simulink model "PhyMtrCtrl"  (R2023b)
settings: Solver=VariableStepAuto  StartTime=0.0  StopTime=10.0  RelTol=1e-3
values from neighbouring files (symbols this model uses):
  B = 0.001889    [MtrCtrl_v01.sldd]    (also in PICal.m; PMSM.m = Simulink.Parameter)
  C_LUT_AngleTable_sng_Null = saveVarsMat.C_LUT_AngleTable_sng_Null    [AngleTable.m]    (also in PMSM.m)
  C_LUT_SinTable_sng_Null = saveVarsMat.C_LUT_SinTable_sng_Null    [AngleTable.m]    (also in PMSM.m)
  C_MATH_OneOverSqrtThree_s32n31_Null = Simulink.Parameter    [PMSM.m]
  C_MATH_Pi_u32n30_Null = Simulink.Parameter    [PMSM.m]
  C_MATH_SqrtThreeOverThree_s32n31_Null = Simulink.Parameter    [PMSM.m]
  C_PMSM_CurQKi_u32n31_null = Simulink.Parameter    [PMSM.m]
  C_PMSM_CurQKp_u32n31_null = Simulink.Parameter    [PMSM.m]
  C_PMSM_Flux_u32n32_Vs = Simulink.Parameter    [PMSM.m]
  Flux = 0.192    [MtrCtrl_v01.sldd]    (also in PICal.m; PMSM.m)
  IBase_A = 2000.0    [MtrCtrl_v01.sldd]    (also in PICal.m = 300; PMSM.m = Simulink.Parameter)
  J = 0.011    [MtrCtrl_v01.sldd]    (also in PICal.m; PMSM.m)
  K_SVM_DefultDuty_s32n31_Null = Simulink.Parameter    [PMSM.m]
  KCCM_VirPosn_flg = 0.0    [MtrCtrl_v01.sldd]    (also in PMSM.m = Simulink.Parameter)
  KCCM_VoltModeEna_Flg = 0.0    [MtrCtrl_v01.sldd]    (also in PMSM.m = Simulink.Parameter)
  Kis = 114583.3333333333    [MtrCtrl_v01.sldd]    (also in PICal.m = 114583.333333; PMSM.m = 114583.333333)
  Kt = 1.1520000000000001    [MtrCtrl_v01.sldd]    (also in PICal.m = 1.152; PMSM.m = 1.152)
  Ld = 80e-6    (= 8e-05)    [FluxweakingGen.m]    (also in IEHB_MAPGenerationtest.m = 6.8e-05; MtrCtrl_v01.sldd = 0.000635; PICal.m = 0.000635; PMSM.m = Simulink.Parameter)
  LPF_coefg = 0.01    [MtrCtrl_v01.sldd]    (also in PMSM.m = Simulink.Parameter)
  Lq = 80e-6    (= 8e-05)    [FluxweakingGen.m]    (also in IEHB_MAPGenerationtest.m = 6e-05; MtrCtrl_v01.sldd = 0.000685; PICal.m = 0.000635; PMSM.m = Simulink.Parameter)
  Ls = 0.000635    [MtrCtrl_v01.sldd]    (also in PICal.m; PMSM.m)
  OneOverUBase_V = Simulink.Parameter    [PMSM.m]
  Pp = 4.0    [MtrCtrl_v01.sldd]    (also in PICal.m = 4; PMSM.m = Simulink.Parameter)
  Rs = 0.03    [FluxweakingGen.m]    (also in MtrCtrl_v01.sldd = 0.05; PICal.m = 0.05; PMSM.m = Simulink.Parameter)
  SecPerRnd = 0.6    [MtrCtrl_v01.sldd]    (also in PMSM.m = Simulink.Parameter)
  sinTable = 0.0015339801862847655 0.0015339807878856412 0.0030679567629659761 0.0030679615757712823 0.0046019261204485705 0.0046019423636569235 0.0061358846491544753 0.0061359231515425647 0.007669828739531097 0.0076699039394282058 0.00920375478205982 0.009203884727313847 0.010737659167264491 0.010737865515199488 0.012271538285719925 0.012271846303085129 0.013805388528060391 0.013805827090970771 0.015339206284    [MtrCtrl_v01.sldd]    (also in SinLut.m = zeros(2,TableSize))
  SMOGain_V = 323.31615074619043    [MtrCtrl_v01.sldd]    (also in PMSM.m = Simulink.Parameter)
  Ts = 0.0001    [MtrCtrl_v01.sldd]    (also in PICal.m; PMSM.m = Simulink.Parameter)
  UBase_V = 600.0    [MtrCtrl_v01.sldd]    (also in PICal.m = 600; PMSM.m = Simulink.Parameter)
  wmBase_rps = 314.15926535897933    [MtrCtrl_v01.sldd]    (also in PICal.m = 314.159265359; PMSM.m = Simulink.Parameter)
undefined symbols (not defined in the file or in its folder): C_PMSM_Ls_pu, C_PMSM_PolePairs_u8_Null, DiscIntNeverNeededParam
libraries: ee_lib x16, simulink x10, nesl_utility x6, spsVoltageMeasurementLib x6, spsCurrentMeasurementLib x3, spsSeriesRLCBranchLib x3, simulink_extras x2, fl_lib x2, sdl_lib x1, eePmsmFwController x1, slpidlib x1, spspowerguiLib x1
(part 1 of 3)
settings Model: Creator=z1486  LastModifiedBy=z1486

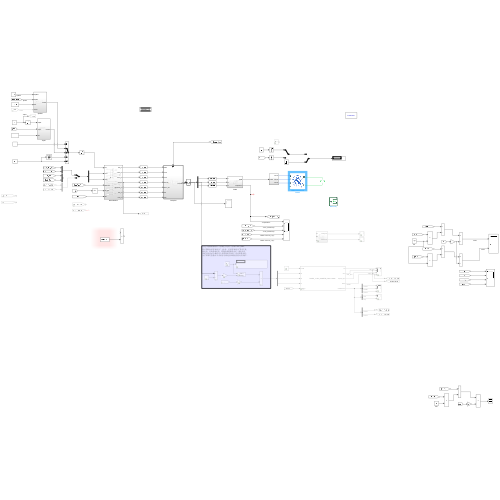
[thumbnail: Simulink's stored preview of the top-level diagram]
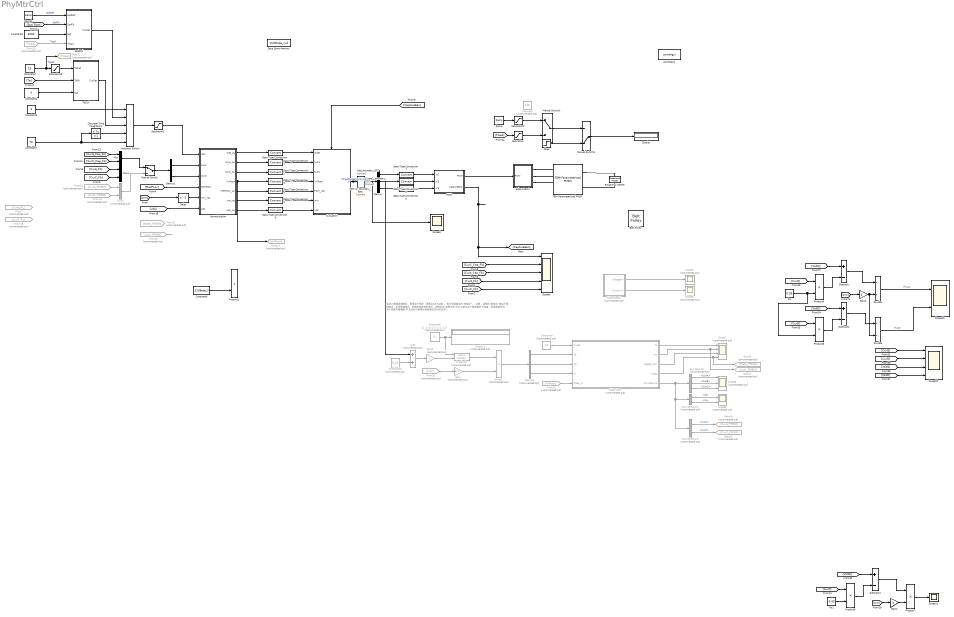
== system PhyMtrCtrl ==
  note: 经过三角载波调制后，再乘这个矩阵，再乘以1/3与Udc，
      | 即可得到真实的“相电压”。(注意，这里的“相电压”其实不是
      | 相电压，应该是端电压，即电机端到地的电压，相电压应
      | 该是正弦)为什么乘以这个矩阵暂时不知道，但结果是对的。
      | 关于结果可查看表“开关状态与相电压和线电压的对应关系”。
  Add : Sum  Commented=on
  Add_boundary_DTC : DataTypeConversion
  Belt Pulley : sdl_lib/Couplings & Drives/Belt Pulley  belt_type=sdl.enum.belt_type.ideal  sheave_ang=30 deg  num_belts=1  model_f_c=sdl.enum.model_centrifugal.off  linear_density=0.6 kg/m  belt_direction=sdl.enum.belt_direction.opposite  breakable=sdl.enum.max_tension.off  F_max=1e5 N  check_tension=sdl.enum.tension_check.off  pulley_moveable=simscape.enum.onoff.off  r_pulley=.15 m  b_pulley=0.001 N*m*s/rad  model_inertia=sdl.enum.model_inertia.off  pulley_mass=0.01 kg  initial_vel=0 m/s  pulley_inertia=0.01 kg*m^2  initial_velocity=0 rad/s  friction_model=sdl.enum.PulleyModel.Modal  initial_state_locked=sdl.enum.initial_lock.unlocked  mu=0.5  mu_static=0.5  mu_kinetic=0.42  phi_wrap=180 deg  v_thr=0.001 m/s  f_thr=0.01 N
      settings: InternalSimscapePortConfiguration="{\"Bottom\":[],\"Left\":[{\"id\":\"S\",\"label\":\"S\",\"type\":\"foundation.mechanical.rotational.rotational\"}],\"Right\":[{\"id\":\"A\",\"label\":\"A\",\"type\":\"foundation.mechanical.translational.translational\"},{\"id\":\"B\",\"label\":\"B\",\"type\":\"foundation.mechanical.translational.translational\"}],\"Top\":[]}"
  Bus Selector : BusSelector  Commented=on  OutputSignals=CurA,CurB,CurC
  Bus Selector2 : BusSelector  Commented=on  OutputSignals=Id,Iq
  Bus Selector3 : BusSelector  Commented=on  OutputSignals=CurA,CurC
  Constant : Constant  Commented=on  Value=100
  Constant10 : Constant  Commented=on  Value=0.25
  Constant2 : Constant  Value=15
  Constant3 : Constant  Value=3
  Constant4 : Constant  Value=5
  Constant5 : Constant  Value=3000
  Constant6 : Constant  Value=1/UBase_V
  Constant7 : Constant  Value=70
  Constant8 : Constant  Commented=on  Value=[2 -1 -1;-1 2 -1;-1 -1 2]
  Constant9 : Constant  Commented=on  Value=10
  CurLpCtrl : Subsystem
      settings: RTWSystemCode=Nonreusable function  RTWFcnNameOpts=Use subsystem name
  Data Store Memory : DataStoreMemory  DataStoreName=VoltMode_null  WriteAfterWriteMsg=warning  ShowAdditionalParam=off
  Data Type Conversion{,1..9} (10 alike) : DataTypeConversion  SaturateOnIntegerOverflow=off  RndMeth=Floor
  Delay : Delay  DelayLength=1
  Demux : Demux  Outputs=3
  Demux1 : Demux  Outputs=2
  Demux2 : Demux  Commented=on  Outputs=3
  Demux_boundary_DTC : DataTypeConversion
  Discrete-Time Integrator2 : DiscreteIntegrator  SampleTime=-1  ICPrevOutput=DiscIntNeverNeededParam  ICPrevScaledInput=DiscIntNeverNeededParam
  Display : Display
  Display1 : Display  Commented=on
  Divide1 : Product  Commented=on  Inputs=**
  Divide2 : Product  Inputs=*/
  Divide3 : Product  Inputs=*/
  FEM-Parameterized PMSM : ee_lib/Electromechanical/Permanent Magnet/FEM-Parameterized PMSM  parameterization=1  winding_type=ee.enum.statorconnection.wye  iVec=[-300, 0, 300] A  xVec=[0, 20, 40, 60] deg  dfluxdiMatrix=0.0002 * ones(3, 4) Wb/A  dfluxdxMatrix=[0, -.16, .16, 0; 0, -.16, .16, 0; 0, -.16, .16, 0] Wb/rad  calculate_torque_matrix=1  TorqueMatrix=zeros(3, 3, 3, 4) N*m  idVec1=[-200, 0, 200] A  iqVec1=[-200, 0, 200] A  LdMatrix=0.0002 * ones(3, 3) H  LqMatrix=0.0002 * ones(3, 3) H  PmMatrix=0.1 * ones(3, 3) Wb  N=4  interp_method=simscape.enum.interpolation.linear  Rs=0.05 Ohm  Ms=0.00002 H  L0=0.00016 H  loss_param=ee.enum.fem_motor.ironLosses.empirical  losses_oc=[0, 0, 0] W  losses_sc=[0, 0, 0] W  f_losses=60 Hz  Isc_losses=95 A  Inertia=0.01 kg*m^2  lam=0 N*m*s/rad  i_d_specify=off  i_d_priority=None  i_d=0 A  i_d_nominal_specify=off  i_d_nominal_unit=A  i_d_nominal_value=1  i_q_specify=off  i_q_priority=None  i_q=0 A  i_q_nominal_specify=off  i_q_nominal_unit=A  i_q_nominal_value=1  torque_specify=off  torque_priority=None  torque=0 N*m  torque_nominal_specify=off  torque_nominal_unit=N*m  torque_nominal_value=1  angular_velocity_specify=off  angular_velocity_priority=High  angular_velocity=0 rpm  angular_velocity_nominal_specify=off  angular_velocity_nominal_unit=rpm  angular_velocity_nominal_value=1  angular_position_specify=off  angular_position_priority=High  angular_position=0 deg  angular_position_nominal_specify=off  angular_position_nominal_unit=deg  angular_position_nominal_value=1  Tmeas=298.15 K  alpha=3.93e-3 1/K  alpha_flux=-0.001 1/K  stator_thermal_mass=100 J/K  stator_initial_temperatures=[298.15, 298.15, 298.15] K  rotor_thermal_mass=200 J/K  rotor_initial_temperature=298.15 K  Rm_percent_rotor=90  Rd_percent_rotor=30  idVec=[-200, 0, 200] A  iqVec=[-200, 0, 200] A  dfluxAdiaMatrix3D=zeros(3, 3, 4) Wb/A  dfluxAdibMatrix3D=zeros(3, 3, 4) Wb/A  dfluxAdicMatrix3D=zeros(3, 3, 4) Wb/A  dfluxAdxMatrix3D=zeros(3, 3, 4) Wb/rad  TorqueMatrix3D=zeros(3, 3, 4) N*m  iaVec=[-200, 0, 200] A  ibVec=[-200, 0, 200] A  icVec=[-200, 0, 200] A  dfluxAdiaMatrix=zeros(3, 3, 3, 4) Wb/A  dfluxAdibMatrix=zeros(3, 3, 3, 4) Wb/A  dfluxAdicMatrix=zeros(3, 3, 3, 4) Wb/A  dfluxAdxMatrix=zeros(3, 3, 3, 4) Wb/rad  param_dq0=ee.enum.fem_motor.fluxTabulationOption.DQcartesian  winding_type_dq0=ee.enum.statorconnection.wye  expose_neutral_port=ee.enum.fem_motor.exposeNeutralPort.no  nPolePairs=4  parks_type=ee.enum.fem_motor.parksType.QleadsD_AphaseToDaxis  idVec2=[-200, 0, 200] A  iqVec2=[-200, 0, 200] A  magVec2=[0, 100, 200] A  betaVec2=[-180, -90, 0, 90, 180] deg  xVec2=[0, 15, 30, 45, 60, 75, 90] deg  fluxD_dq0=zeros(3, 3, 7) Wb  fluxQ_dq0=zeros(3, 3, 7) Wb  fluxA_dq0=zeros(3, 3, 7) Wb  Torque_dq0=ones(3, 3, 7) N*m  fluxD_IBX=zeros(3, 5, 7) Wb  fluxQ_IBX=zeros(3, 5, 7) Wb  fluxA_IBX=zeros(3, 5, 7) Wb  Torque_IBX=zeros(3, 5, 7) N*m  rotorLossCoeff_k_h_DQ=zeros(3, 3) W/Hz  rotorLossCoeff_k_J_DQ=zeros(3, 3) W/Hz^2  rotorLossCoeff_k_ex_DQ=zeros(3, 3) W/Hz^(3/2)  rotorLossCoeff_k_h_IB=zeros(3, 5) W/Hz  rotorLossCoeff_k_J_IB=zeros(3, 5) W/Hz^2  rotorLossCoeff_k_ex_IB=zeros(3, 5) W/Hz^(3/2)  statorLossCoeff_k_h_DQ=zeros(3, 3) W/Hz  statorLossCoeff_k_J_DQ=zeros(3, 3) W/Hz^2  statorLossCoeff_k_ex_DQ=zeros(3, 3) W/Hz^(3/2)  statorLossCoeff_k_h_IB=zeros(3, 5) W/Hz  statorLossCoeff_k_J_IB=zeros(3, 5) W/Hz^2  statorLossCoeff_k_ex_IB=zeros(3, 5) W/Hz^(3/2)  wVec=[1000, 2000] rpm  rotorLossTable_DQ=zeros(3, 3, 2) W  rotorLossTable_IB=zeros(3, 5, 2) W  statorLossTable_DQ=zeros(3, 3, 2) W  statorLossTable_IB=zeros(3, 5, 2) W  electrical_torque_before_iron_losses_specify=off  electrical_torque_before_iron_losses_priority=None  electrical_torque_before_iron_losses=0 N*m  electrical_torque_before_iron_losses_nominal_specify=off  electrical_torque_before_iron_losses_nominal_unit=N*m  electrical_torque_before_iron_losses_nominal_value=1  Qrotor_specify=off  Qrotor_priority=None  Qrotor=0 J/s  Qrotor_nominal_specify=off  Qrotor_nominal_unit=J/s  Qrotor_nominal_value=1  Qstator_specify=off  Qstator_priority=None  Qstator=0 J/s  Qstator_nominal_specify=off  Qstator_nominal_unit=J/s  Qstator_nominal_value=1
      settings: InternalSimscapePortConfiguration="{\"Bottom\":[],\"Left\":[{\"id\":\"a\",\"label\":\"a\",\"type\":\"foundation.electrical.electrical\"},{\"id\":\"b\",\"label\":\"b\",\"type\":\"foundation.electrical.electrical\"},{\"id\":\"c\",\"label\":\"c\",\"type\":\"foundation.electrical.electrical\"},{\"id\":\"n\",\"label\":\"n\",\"type\":\"foundation.electrical.electrical\"}],\"Right\":[{\"id\":\"R\",\"label\":\"R\",\"type\":\"foundation.mechanical.rotational.rotational\"},{\"id\":\"C\",\"label\":\"C\",\"type\":\"foundation.mechanical.rotational.rotational\"}],\"Top\":[]}"
  From10 : From  Commented=on  GotoTag=Tload
  From18 : From  Commented=on  GotoTag=CurC_RL
  From20 : From  Commented=on  GotoTag=Udc
  From22 : From  Commented=on  GotoTag=VirPosn
  From23 : From  Commented=on  GotoTag=CurA_PMSM
  From24 : From  Commented=on  GotoTag=CurC_PMSM
  From25 : From  Commented=on  GotoTag=theta_PMSM
  From26 : From  Commented=on  GotoTag=wm_PMSM
  From7 : From  Commented=on  GotoTag=CurA_RL
  Gain : Gain  Commented=on  Gain=1/3
  Gain2 : Gain  Commented=on  Gain=-1
  Gain3 : Gain  Gain=4
  Gain4 : Gain  Gain=4
  Goto11 : Goto  Commented=on  GotoTag=Tload
  Goto13 : Goto  Commented=on  GotoTag=VirPosn
  Goto14 : Goto  Commented=on  GotoTag=CurA_PMSM
  Goto15 : Goto  Commented=on  GotoTag=CurC_PMSM
  Goto16 : Goto  Commented=on  GotoTag=theta_PMSM
  Goto17 : Goto  Commented=on  GotoTag=wm_PMSM
  Manual Switch : ManualSwitch
  Manual Switch1 : ManualSwitch
  Manual Switch3 : ManualSwitch  CurrentSetting=0
  Multiport Switch : MultiPortSwitch  Inputs=4  SaturateOnIntegerOverflow=off  InputSameDT=off
  Mux : Mux  Inputs=2
  Mux1 : Mux  Inputs=2
  Mux2 : Mux  Commented=on  Inputs=2
  Normalization : Subsystem
  PWM : Subsystem
  Product{2,4,6..8} (5 alike) : Product
  Product3 : Product  Commented=on  Multiplication=Matrix(*)  RndMeth=Zero
  Ramp : simulink/Sources/Ramp  slope=30  start=0  InitialOutput=0
  Ramp1 : simulink/Sources/Ramp  slope=2000  start=0  InitialOutput=0
  Rotational Inerter : fl_lib/Mechanical/Rotational Elements/Rotational Inerter  B=1 kg*m^2  w_specify=off  w_priority=High  w=0 rad/s  w_nominal_specify=off  w_nominal_unit=rad/s  w_nominal_value=1  t_specify=off  t_priority=None  t=0 N*m  t_nominal_specify=off  t_nominal_unit=N*m  t_nominal_value=1
      settings: InternalSimscapePortConfiguration="{\"Bottom\":[],\"Left\":[{\"id\":\"R\",\"label\":\"R\",\"type\":\"foundation.mechanical.rotational.rotational\"}],\"Right\":[{\"id\":\"C\",\"label\":\"C\",\"type\":\"foundation.mechanical.rotational.rotational\"}],\"Top\":[]}"
  Rs : Constant  Value=0.05
  Rs1 : Constant  Value=0.05
  Saturation : Saturate  UpperLimit=200  LowerLimit=-5
  Saturation1 : Saturate  UpperLimit=220
  Saturation2 : Saturate  UpperLimit=30
  Saturation3 : Saturate  UpperLimit=11
  Scope10 : Scope  NumInputPorts=2
  Scope11 : Scope
  Scope12 : Scope  NumInputPorts=4
  Scope2 : Scope
  Scope2_boundary_DTC : DataTypeConversion
  Scope4 : Scope  NumInputPorts=5
  Scope5 : Scope  Commented=on
  Scope6 : Scope  Commented=on
  Scope7 : Scope  Commented=on  NumInputPorts=4
  Scope8 : Scope  Commented=on  NumInputPorts=3
  Scope9 : Scope  Commented=on  NumInputPorts=2
  SpdCtrl : Subsystem
  Step : Step  Time=0.01  After=100  SampleTime=0
  Subsystem : Subsystem  Commented=on  mask{Ld=Ls, Lq=Ls, Rs=Rs, Flux=Flux, J=J, B=B, MaxSpd=10000, Pp=4, PosnSelector=0}
      mask prompts: Rs "Phase Resisitor"; Flux "Flux Linkage"; J "Inertia"; B "Viscous damping"; MaxSpd "Max speed set"; Pp "Pole pairs"; PosnSelector "VirPosnEna"
      mask Display: disp("PMSM_111Nm_3000RPM_560V-129Nm")
  Subsystem1 : Subsystem
  Subsystem2 : Subsystem  Commented=on
  Subtract : Sum  Inputs=+-
  Subtract1 : Sum  Inputs=+-
  Subtract2 : Sum  Inputs=+-
  TqCtrl : Subsystem
  powergui1 : spspowerguiLib/powergui  Priority=1  SimulationMode=Continuous  SampleTime=50e-6  frequency=60  Iterations=50  frequencyindice=60  Pbase=100e6  ErrMax=1e-4  UnitsV=kV  UnitsW=MW  buscounter=0  FunctionMessages=off  echomessages=off  EnableUseOfTLC=off  CurrentSourceSwitches=off  DisableSnubberDevices=off  DisableRonSwitches=off  DisableVfSwitches=off  DisplayEquations=off  AutomaticDiscreteSolvers=off  SolverType=Tustin/Backward Euler (TBE)  Interpol=off  ExternalGateDelay=off  methode=off  Ts=100  x0status=blocks  SPID=on  SwTol=0  HookPort=off  NonlinearTolerance=1e-4  nMaxIteration=100  ContinueOnMaxIteration=off  RestoreLinks=warning  ResistiveCurrentMeasurement=off  Frange=[0:2:500]  Ylog=off  Xlog=on  ShowGrid=off  save=off  variable=ZData  structure=0  ZoomFFT=off  StartTime=0.0  cycles=1  DisplayStyle=1  fundamental=60  FreqAxis=off  MaxFrequency=1000  frequencyindicesteady=1  RmsSteady=1  display=off
  wires:
  Subtract/1 -> Divide2/1
  [VoltD] -> Subtract2/1
  [CurD] -> Product8/1
  [wm] -> Gain4/1
  [CurQ] -> Product6/1
  Rs1/1 -> Product6/2
  Gain4/1 -> Product7/2
  Product6/1 -> Subtract1/2
  Subtract1/1 -> Product7/1
  [wm] -> Gain3/1
  [VoltQ] -> Subtract/1
  [VoltQ] -> Scope12/3
  [CurD] -> Scope12/2
  [VoltD] -> Scope12/4
  Rs/1 -> Product8/2, Product4/2
  [CurQ] -> Scope12/1
  From26/1 -> ?
  Data Type Conversion5/1 -> CurLpCtrl/6(wm)
  Saturation2/1 -> Manual Switch1/1
  Gain2/1 -> Product3/2
  Scope2_boundary_DTC/1 -> Scope2/1
  Normalization/4(VirPosn) -> Data Type Conversion3/1, Goto13/1
  Bus Selector/2 -> Scope8/2  "<CurB>"
  Data Type Conversion7/1 -> PWM/1(In1)
  Data Type Conversion9/1 -> PWM/3(In5)
  Saturation1/1 -> Normalization/1(Iset)
  Add_boundary_DTC/1 -> Add/1
  Data Type Conversion4/1 -> CurLpCtrl/5(Posn_rad)
  Data Type Conversion2/1 -> CurLpCtrl/3(CurC)
  Data Type Conversion6/1 -> CurLpCtrl/7(Udc)
  Data Type Conversion3/1 -> CurLpCtrl/4(VirPosn)
  Subtract2/1 -> Divide3/1
  [CaptureEan] -> CurLpCtrl/Trigger
  Data Type Conversion/1 -> CurLpCtrl/1(IsSet)
  Constant3/1 -> Multiport Switch/1
  Normalization/1(Iset_pu) -> Data Type Conversion/1
  CurLpCtrl/1(S) -> Add_boundary_DTC/1, Demux_boundary_DTC/1, Scope2_boundary_DTC/1  "ThreePhaseDutyCycle"
  Normalization/2(CurA_pu) -> Data Type Conversion1/1
  Data Type Conversion1/1 -> CurLpCtrl/2(CurA)
  Ramp/1 -> Saturation2/1
  Subsystem/2(wm) -> Goto17/1, Scope7/2
  Bus Selector/3 -> Scope8/3  "<CurC>"
  Demux2/1 -> Subsystem/2(Va)
  From23/1 -> Mux2/1
  Discrete-Time Integrator2/1 -> Multiport Switch/4
  [Tload] -> Saturation/1
  Normalization/6(wm_pu) -> Data Type Conversion5/1
  [wm] -> Delay/1
  From24/1 -> Mux2/2
  Demux2/2 -> Subsystem/3(Vb)
  From22/1 -> Subsystem/5(Theta_In)
  Add/1 -> Gain2/1
  Subsystem/4(theta) -> Goto16/1, Scope7/4
  Bus Selector3/2 -> Goto15/1  "<CurC>"
  [MecPosn] -> Normalization/4(MecPosn)
  SpdCtrl/1(CurSet) -> Multiport Switch/2
  Bus Selector3/1 -> Goto14/1  "<CurA>"
  Mux2/1 -> Manual Switch/2
  Constant10/1 -> Add/2
  From10/1 -> SpdCtrl/4(Tload)  "Tload"
  Subsystem/3(Speed_rpm) -> Scope7/3
  Bus Selector2/1 -> Scope9/1  "<Id>"
  Manual Switch3/1 -> Display/1
  Delay/1 -> Normalization/5(wm_rps)
  Normalization/3(CurC_pu) -> Data Type Conversion2/1
  [CurC_Fb] -> Mux1/2
  Constant8/1 -> Product3/1, Display1/1
  [VoltQ] -> Subtract1/1
  Data Type Conversion8/1 -> PWM/2(In3)
  Demux2/3 -> Subsystem/4(Vc)
  Saturation3/1 -> TqCtrl/1(TqRef)
  Constant9/1 -> Subsystem/1(TLoad)
  Bus Selector/1 -> Scope8/1  "<CurA>"
  Subsystem/1(Te) -> Scope7/1
  Bus Selector2/2 -> Scope9/2  "<Iq>"
  Product7/1 -> Scope11/1
  Subsystem/5(CurMaesure) -> Bus Selector/1, Bus Selector3/1, Bus Selector2/1
  Product8/1 -> Subtract2/2
  Constant7/1 -> Discrete-Time Integrator2/1, Multiport Switch/5
  Saturation/1 -> Manual Switch1/2
  Normalization/7(Udc_pu) -> Data Type Conversion6/1
  Subsystem2/1(Voltage M) -> Scope5/1
  Gain3/1 -> Divide3/2, Divide2/2
  Demux/1 -> Data Type Conversion7/1
  Subsystem2/2(Current M) -> Scope6/1
  Multiport Switch/1 -> Saturation1/1
  [Udc] -> Normalization/6(Udc)
  Demux1/2 -> Normalization/3(CurC)
  [Spd_Rpm] -> SpdCtrl/2(SpdFb)  "SpdFb"
  Constant5/1 -> SpdCtrl/3(Sat)
  TqCtrl/1(CurSet) -> Multiport Switch/3
  [CurA_Cap_Fb] -> Mux/1
  Mux/1 -> Manual Switch/1
  Constant4/1 -> TqCtrl/3(Sat)
  Demux_boundary_DTC/1 -> Demux/1
  Normalization/5(MecPosn_pu) -> Data Type Conversion4/1
  Manual Switch/1 -> Demux1/1
  Constant6/1 -> Product2/2
  [Te] -> TqCtrl/2(TqFb)
  Constant2/1 -> Goto11/1, Saturation3/1  "TqRef"
  [CurC_Fb] -> Scope4/5
  Step/1 -> Manual Switch3/2
  [CurA_Cap_Fb] -> Scope4/3
  Demux/2 -> Data Type Conversion8/1
  Divide1/1 -> Demux2/1
  Demux/3 -> Data Type Conversion9/1
  [CurC_Cap_Fb] -> Scope4/2
  Ramp1/1 -> SpdCtrl/1(SpdRef)  "SpdRef"
  Demux1/1 -> Normalization/2(CurA)
  PWM/2(CaptureEna) -> [CaptureEan], Scope4/1
  Product3/1 -> Divide1/1
  Gain/1 -> Divide1/2
  [CurA_Fb] -> Scope4/4
  Divide3/1 -> Scope10/2  "FluxD"
  From20/1 -> Gain/1
  Manual Switch1/1 -> Manual Switch3/1
  Product4/1 -> Subtract/2
  [CurA_Fb] -> Mux1/1
  [CurC_Cap_Fb] -> Mux/2
  Divide2/1 -> Scope10/1  "FluxQ"
  PWM/1(PWM) -> Subsystem1/1(PWM)
  [CurQ] -> Product4/1
  connections:
  Subsystem1/RConn2 -- FEM-Parameterized PMSM/LConn2
  Subsystem1/RConn1 -- FEM-Parameterized PMSM/LConn1
  Subsystem1/RConn3 -- FEM-Parameterized PMSM/LConn3
  FEM-Parameterized PMSM/RConn1 -- Rotational Inerter/LConn1
  Rotational Inerter/RConn1 -- FEM-Parameterized PMSM/RConn2

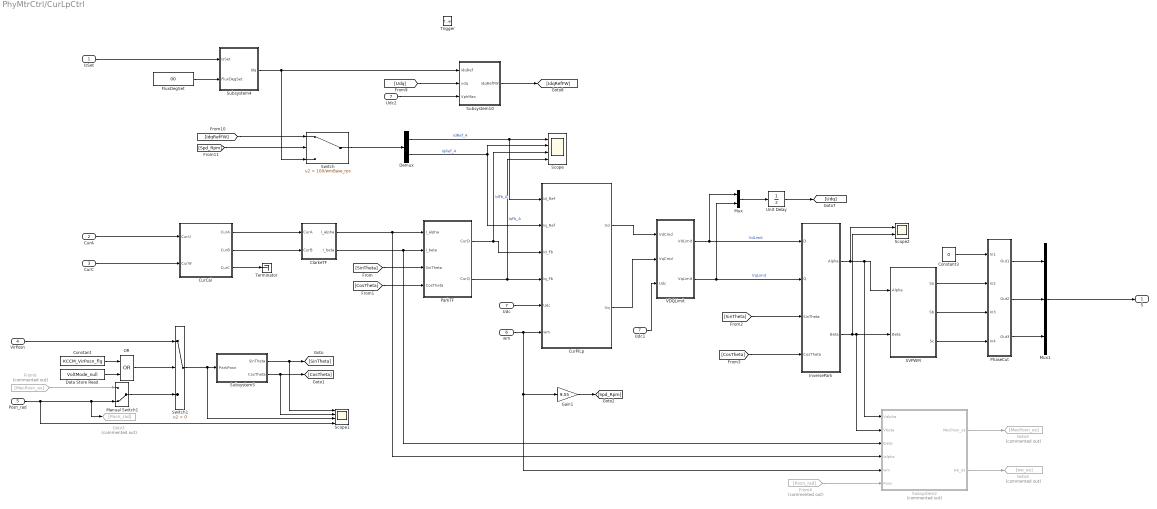
== system PhyMtrCtrl/CurLpCtrl ==
  IsSet : Inport  OutDataTypeStr=fixdt(1,32,31)
  CurA : Inport  Port=2  OutDataTypeStr=fixdt(1,32,31)
  CurC : Inport  Port=3  OutDataTypeStr=fixdt(1,32,31)
  VirPosn : Inport  Port=4  OutDataTypeStr=fixdt(1,32,28)
  Posn_rad : Inport  Port=5  OutDataTypeStr=fixdt(1,32,28)
  wm : Inport  Port=6  OutDataTypeStr=fixdt(1,32,31)
  Udc : Inport  Port=7  OutDataTypeStr=fixdt(0,32,32)
  Trigger : TriggerPort  VariantControl=(inherit)  PortDimensions=1
  ClarkeTF : Subsystem
  Constant : Constant  Value=KCCM_VirPosn_flg
  Constant3 : Constant  Value=0  OutDataTypeStr=fixdt(1,32,4)
  CurCal : Subsystem
  CurPILp : Subsystem
  Data Store Read : DataStoreRead  DataStoreName=VoltMode_null  IndexOptions=Index vector (dialog)  Indices=1  OutputSizes=1
  Demux : Demux  Outputs=2
  FluxDegSet : Constant  Value=00  OutDataTypeStr=fixdt(1,32,4)
  From4 : From  Commented=on  GotoTag=Posn_rad
  From6 : From  Commented=on  GotoTag=MecPosn_es
  Gain1 : Gain  Gain=9.55  OutDataTypeStr=fixdt(0,32,30)
  Goto3 : Goto  Commented=on  GotoTag=Posn_rad
  Goto4 : Goto  Commented=on  GotoTag=we_es
  Goto5 : Goto  Commented=on  GotoTag=MecPosn_es
  InversePark : Subsystem
  Manual Switch1 : ManualSwitch  CurrentSetting=0
  Mux : Mux  Inputs=2
  Mux1 : Mux  Inputs=3
  OR : Logic  Operator=OR  AllPortsSameDT=off  OutDataTypeStr=boolean
  ParkTF : Subsystem
  PhaseCut : Subsystem
  SVPWM : Subsystem
  Scope : Scope  NumInputPorts=4
  Scope1 : Scope  NumInputPorts=4
  Scope2 : Scope  NumInputPorts=2
  Subsystem10 : Subsystem
  Subsystem2 : Subsystem  Commented=on
  Subsystem4 : Subsystem
  Subsystem5 : Subsystem
  Switch : Switch  Criteria=u2 > Threshold  Threshold=100/wmBase_rps  OutDataTypeStr=fixdt(1,32,31)  SaturateOnIntegerOverflow=off  InputSameDT=off
  Switch1 : Switch  Criteria=u2 > Threshold  OutDataTypeStr=fixdt(1,32,28)  SaturateOnIntegerOverflow=off  InputSameDT=off
  Terminator : Terminator
  Udc1 : InportShadow  Port=7  OutDataTypeStr=fixdt(0,32,32)
  Udc2 : InportShadow  Port=7  OutDataTypeStr=fixdt(0,32,32)
  Unit Delay : UnitDelay  SampleTime=-1  HasFrameUpgradeWarning=on
  VDQLimit : Subsystem
  S : Outport
  wires:
  Subsystem10/1(idqRefFW) -> [IdqRefFW]
  Demux/1 -> CurPILp/1(Id_Ref), Scope/1  "IdRef_A"
  [IdqRefFW] -> Switch/1
  [SinTheta] -> InversePark/3(SinTheta)
  Mux/1 -> Unit Delay/1
  ParkTF/2(CurQ) -> Scope/4, CurPILp/4(Iq_Fb)  "IqFb_A"
  VirPosn/1 -> Switch1/1
  CurPILp/1(Vd) -> VDQLimit/1(VdCmd)
  CurA/1 -> CurCal/1(CurU)
  CurPILp/2(Vq) -> VDQLimit/2(VqCmd)
  Switch/1 -> Demux/1
  Subsystem5/1(SinTheta) -> Scope1/1, [SinTheta]
  [Spd_Rpm] -> Switch/2
  Subsystem5/2(CosTheta) -> Scope1/2, [CosTheta]
  ParkTF/1(CurD) -> Scope/3, CurPILp/3(Id_Fb)  "IdFb_A"
  [Udq] -> Subsystem10/2(vdq)
  CurCal/1(CurA) -> ClarkeTF/1(CurA)
  ClarkeTF/2(I_beta) -> Subsystem2/3(Ibeta), ParkTF/2(I_beta)
  ClarkeTF/1(I_alpha) -> Subsystem2/4(Ialpha), ParkTF/1(I_alpha)
  CurC/1 -> CurCal/2(CurW)
  FluxDegSet/1 -> Subsystem4/2(FluxDegSet)
  [CosTheta] -> ParkTF/4(CosTheta)
  Mux1/1 -> S/1
  [CosTheta] -> InversePark/4(CosTheta)
  [SinTheta] -> ParkTF/3(SinTheta)
  InversePark/2(Beta) -> Scope2/2, Subsystem2/2(Vbeta), SVPWM/2(Beta)
  Demux/2 -> CurPILp/2(Iq_Ref), Scope/2  "IqRef_A"
  CurCal/2(CurB) -> ClarkeTF/2(CurB)
  Manual Switch1/1 -> Switch1/3
  wm/1 -> CurPILp/6(wm), Subsystem2/5(wm), Gain1/1
  Gain1/1 -> [Spd_Rpm]
  Subsystem4/1(Idq) -> Switch/3, Subsystem10/1(idqRef)
  VDQLimit/1(VdLimit) -> Mux/1, InversePark/1(D)  "VdLimit"
  VDQLimit/2(VqLimit) -> Mux/2, InversePark/2(Q)  "VqLimit"
  Udc/1 -> CurPILp/5(Udc)
  Udc2/1 -> Subsystem10/3(VphMax)
  Unit Delay/1 -> [Udq]
  Constant3/1 -> PhaseCut/1(In1)
  SVPWM/1(Sa) -> PhaseCut/2(In2)
  SVPWM/2(Sb) -> PhaseCut/3(In3)
  SVPWM/3(Sc) -> PhaseCut/4(In4)
  PhaseCut/1(Out1) -> Mux1/1
  PhaseCut/2(Out2) -> Mux1/2
  PhaseCut/3(Out3) -> Mux1/3
  IsSet/1 -> Subsystem4/1(IsSet)
  Udc1/1 -> VDQLimit/3(Udc)
  InversePark/1(Alpha) -> Scope2/1, Subsystem2/1(Valpha), SVPWM/1(Alpha)
  From4/1 -> Subsystem2/6(Posn)
  Subsystem2/2(we_es) -> Goto4/1
  Subsystem2/1(MecPosn_es) -> Goto5/1
  Posn_rad/1 -> Scope1/4, Manual Switch1/2, Goto3/1
  From6/1 -> Manual Switch1/1
  Switch1/1 -> Scope1/3, Subsystem5/1(ParkPosn)
  Constant/1 -> OR/1
  Data Store Read/1 -> OR/2
  OR/1 -> Switch1/2
  CurCal/3(CurC) -> Terminator/1

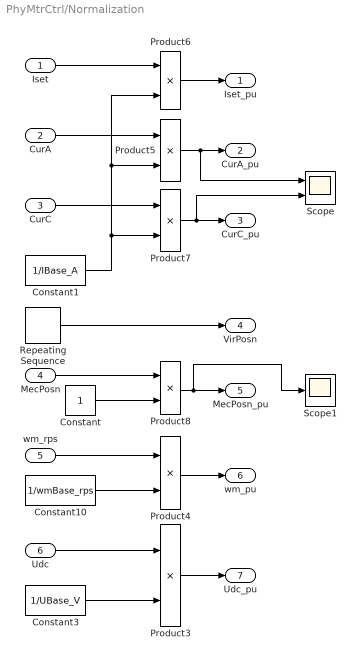
== system PhyMtrCtrl/Normalization ==
  Iset : Inport
  CurA : Inport  Port=2
  CurC : Inport  Port=3
  MecPosn : Inport  Port=4
  wm_rps : Inport  Port=5
  Udc : Inport  Port=6
  Constant : Constant
  Constant1 : Constant  Value=1/IBase_A
  Constant10 : Constant  Value=1/wmBase_rps
  Constant3 : Constant  Value=1/UBase_V
  Product{3..8} (6 alike) : Product
  Repeating Sequence : simulink/Sources/Repeating Sequence  rep_seq_t=[0 SecPerRnd]  rep_seq_y=[0 2*pi]
  Scope : Scope  NumInputPorts=2
  Scope1 : Scope
  Iset_pu : Outport
  CurA_pu : Outport  Port=2
  CurC_pu : Outport  Port=3
  VirPosn : Outport  Port=4
  MecPosn_pu : Outport  Port=5
  wm_pu : Outport  Port=6
  Udc_pu : Outport  Port=7
  wires:
  Product6/1 -> Iset_pu/1
  Product4/1 -> wm_pu/1
  Constant1/1 -> Product6/2, Product5/2, Product7/2
  Product3/1 -> Udc_pu/1
  Constant10/1 -> Product4/2
  Constant3/1 -> Product3/2
  MecPosn/1 -> Product8/1
  CurC/1 -> Product7/1
  Product5/1 -> Scope/1, CurA_pu/1
  Product7/1 -> Scope/2, CurC_pu/1
  CurA/1 -> Product5/1
  Udc/1 -> Product3/1
  Product8/1 -> Scope1/1, MecPosn_pu/1
  wm_rps/1 -> Product4/1
  Constant/1 -> Product8/2
  Repeating Sequence/1 -> VirPosn/1
  Iset/1 -> Product6/1

== system PhyMtrCtrl/PWM ==
  In1 : Inport
  In3 : Inport  Port=2
  In5 : Inport  Port=3
  Compare To Constant : simulink/Logic and Bit Operations/Compare To Constant  relop=<=  const=0.003  OutDataTypeStr=boolean
  Gain : Gain  Gain=0.3
  Gain1 : Gain  Gain=0.6
  Mux : Mux  Inputs=6
  NOT : Logic  Operator=NOT  AllPortsSameDT=off  OutDataTypeStr=boolean
  NOT1 : Logic  Operator=NOT  AllPortsSameDT=off  OutDataTypeStr=boolean
  NOT2 : Logic  Operator=NOT  AllPortsSameDT=off  OutDataTypeStr=boolean
  Relational Operator : RelationalOperator  Operator=<=  OutDataTypeStr=boolean  RndMeth=Simplest  InputSameDT=off
  Relational Operator1 : RelationalOperator  Operator=<=  OutDataTypeStr=boolean  RndMeth=Simplest  InputSameDT=off
  Relational Operator2 : RelationalOperator  Operator=<=  OutDataTypeStr=boolean  RndMeth=Simplest  InputSameDT=off
  Repeating Sequence : simulink/Sources/Repeating Sequence  rep_seq_t=[0 Ts/2 Ts]  rep_seq_y=[0 0.5 0]
  Scope : Scope  NumInputPorts=4
  Scope2 : Scope  NumInputPorts=6
  PWM : Outport
  CaptureEna : Outport  Port=2
  wires:
  Relational Operator1/1 -> NOT1/1, Gain1/1, Mux/3  "PWM_VH"
  Relational Operator/1 -> NOT/1, Scope2/2, Mux/1  "PWM_UH"
  Repeating Sequence/1 -> Compare To Constant/1, Scope/1, Relational Operator1/2, Scope2/3, Relational Operator/2, Relational Operator2/2  "PWM_Cnt"
  Relational Operator2/1 -> NOT2/1, Gain/1, Mux/5  "PWM_WH"
  NOT1/1 -> Mux/4
  NOT/1 -> Mux/2
  NOT2/1 -> Mux/6
  Mux/1 -> PWM/1
  In5/1 -> Scope/4, Relational Operator2/1  "Duty_W"
  Compare To Constant/1 -> Scope2/4, CaptureEna/1  "CaptureEna"
  Gain/1 -> Scope2/6  "PWM_WH"
  Gain1/1 -> Scope2/5  "PWM_VH"
  In1/1 -> Scope2/1, Relational Operator/1, Scope/2  "Duty_U"
  In3/1 -> Scope/3, Relational Operator1/1  "Duty_V"

== system PhyMtrCtrl/SpdCtrl ==
  SpdRef : Inport
  SpdFb : Inport  Port=2
  Sat : Inport  Port=3
  Tload : Inport  Port=4
  Add : Sum
  Gain : Gain  Gain=23
  Saturation : Saturate  UpperLimit=2000  LowerLimit=-2800
  Scope1 : Scope
  Scope5 : Scope  NumInputPorts=2
  Subsystem1 : Subsystem
  CurSet : Outport
  wires:
  Subsystem1/1(PIOut) -> Scope1/1, Add/1  "SpdPIOut"
  SpdFb/1 -> Subsystem1/2(Fbk), Scope5/2
  SpdRef/1 -> Saturation/1
  Gain/1 -> Add/2
  Sat/1 -> Subsystem1/3(Sat)
  Add/1 -> CurSet/1
  Tload/1 -> Gain/1
  Saturation/1 -> Scope5/1, Subsystem1/1(Ref)

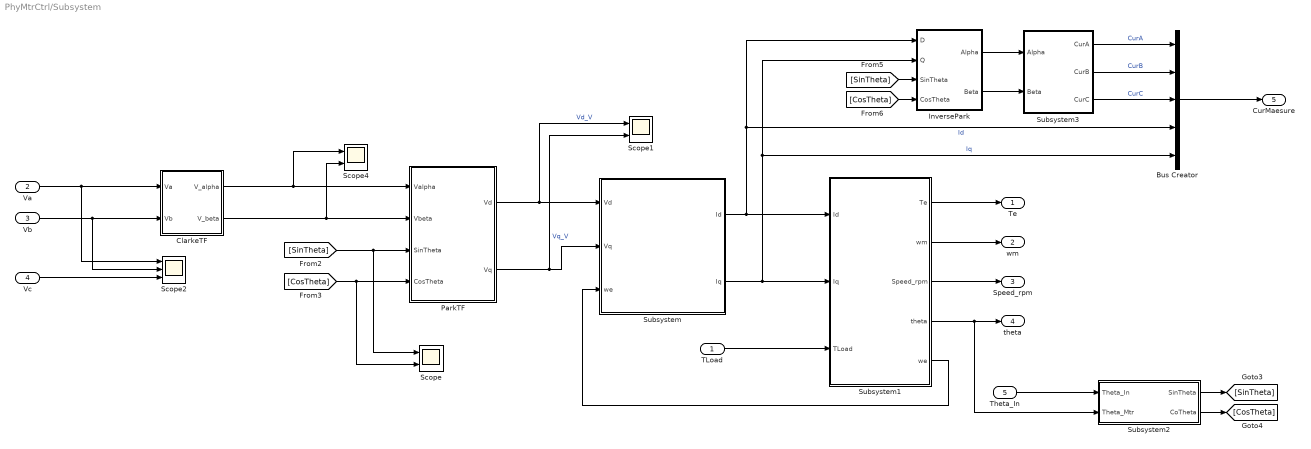
== system PhyMtrCtrl/Subsystem ==
  TLoad : Inport
  Va : Inport  Port=2
  Vb : Inport  Port=3
  Vc : Inport  Port=4
  Theta_In : Inport  Port=5
  Bus Creator : BusCreator  Inputs=5
  ClarkeTF : Subsystem
  InversePark : Subsystem
  ParkTF : Subsystem
  Scope : Scope  NumInputPorts=2
  Scope1 : Scope  NumInputPorts=2
  Scope2 : Scope  NumInputPorts=3
  Scope4 : Scope  NumInputPorts=2
  Subsystem : Subsystem
  Subsystem1 : Subsystem
  Subsystem2 : Subsystem
  Subsystem3 : Subsystem
  Te : Outport
  wm : Outport  Port=2
  Speed_rpm : Outport  Port=3
  theta : Outport  Port=4
  CurMaesure : Outport  Port=5
  wires:
  Va/1 -> Scope2/1, ClarkeTF/1(Va)
  Vb/1 -> Scope2/2, ClarkeTF/2(Vb)
  ClarkeTF/1(V_alpha) -> Scope4/1, ParkTF/1(Valpha)
  ClarkeTF/2(V_beta) -> Scope4/2, ParkTF/2(Vbeta)
  [SinTheta] -> Scope/1, ParkTF/3(SinTheta)
  [CosTheta] -> Scope/2, ParkTF/4(CosTheta)
  ParkTF/1(Vd) -> Scope1/1, Subsystem/1(Vd)  "Vd_V"
  ParkTF/2(Vq) -> Scope1/2, Subsystem/2(Vq)  "Vq_V"
  Subsystem/2(Iq) -> InversePark/2(Q), Bus Creator/5, Subsystem1/2(Iq)  "Iq"
  Subsystem/1(Id) -> InversePark/1(D), Bus Creator/4, Subsystem1/1(Id)  "Id"
  Subsystem1/5(we) -> Subsystem/3(we)
  Subsystem2/1(SinTheta) -> [SinTheta]
  Subsystem2/2(CoTheta) -> [CosTheta]
  TLoad/1 -> Subsystem1/3(TLoad)
  Subsystem1/1(Te) -> Te/1
  Subsystem1/2(wm) -> wm/1
  Subsystem1/3(Speed_rpm) -> Speed_rpm/1
  [SinTheta] -> InversePark/3(SinTheta)
  [CosTheta] -> InversePark/4(CosTheta)
  InversePark/1(Alpha) -> Subsystem3/1(Alpha)
  InversePark/2(Beta) -> Subsystem3/2(Beta)
  Subsystem3/1(CurA) -> Bus Creator/1  "CurA"
  Subsystem3/3(CurC) -> Bus Creator/3  "CurC"
  Subsystem3/2(CurB) -> Bus Creator/2  "CurB"
  Bus Creator/1 -> CurMaesure/1
  Subsystem1/4(theta) -> Subsystem2/2(Theta_Mtr), theta/1
  Theta_In/1 -> Subsystem2/1(Theta_In)
  Vc/1 -> Scope2/3

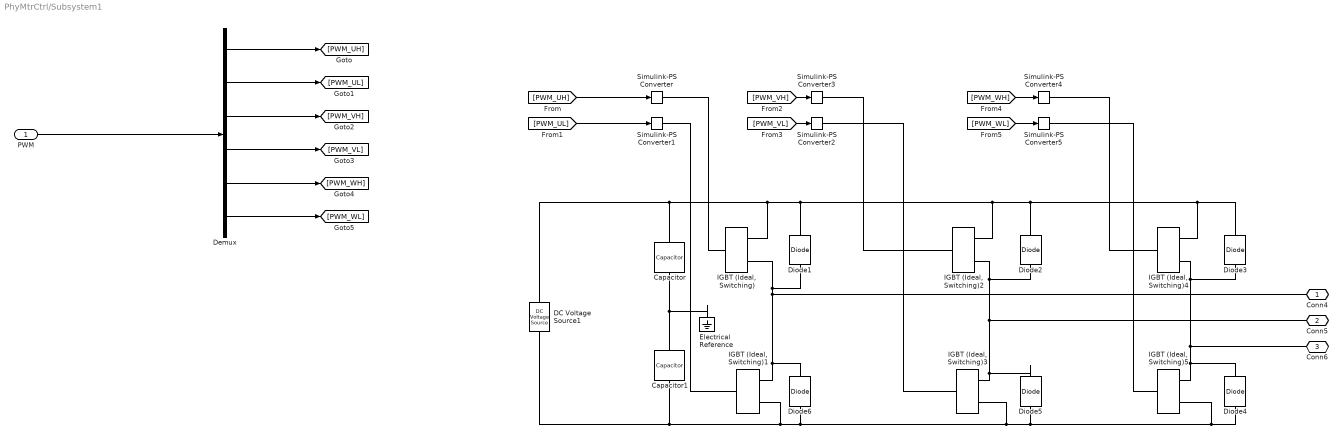
== system PhyMtrCtrl/Subsystem1 ==
  PWM : Inport
  Capacitor : ee_lib/Passive/Capacitor  cap_option=ee.enum.passive.capacitor.capOption.table  c=1e-6 F  Cvec=[0.3125, 6.2500e-02] uF  Vvec=[0, 600] V  CV_table_symmetry=ee.enum.passive.capacitor.tableSymmetry.yes  f_vec=[1, 10] kHz  DFext_vec=[.8, 1.2]  enable_C_tol=ee.enum.toleranceApplication.none  averaging_period=0 s  C_tol=5  tol_distribution=ee.enum.toleranceDistribution.uniform  nSigma=4  r=1e-6 Ohm  g=0 1/Ohm  enable_operating_limits=ee.enum.enable.no  operating_limit_action=ee.enum.passive.reportOpLim.warn  max_working_voltage_range=[-25, 25] V  power_rating=1 W  enable_faults=ee.enum.enable.no  fault_action=simscape.enum.assert.action.none  Cscale_faulted=100  R_faulted=1e-3 Ohm  G_faulted=0 1/Ohm  tau_fault=1e-3 s  fault_trigger=ee.enum.faults.faultTrigger.temporal  t_fault=1 s  max_permissible_voltage_range=[-100, 100] V  t_fail_on_voltage=1 s  i_specify=off  i_priority=None  i=0 A  i_nominal_specify=off  i_nominal_unit=A  i_nominal_value=1  v_specify=off  v_priority=None  v=0 V  v_nominal_specify=off  v_nominal_unit=V  v_nominal_value=1  vc_specify=off  vc_priority=High  vc=0 V  vc_nominal_specify=off  vc_nominal_unit=V  vc_nominal_value=1
  Capacitor1 : ee_lib/Passive/Capacitor  cap_option=ee.enum.passive.capacitor.capOption.table  c=1e-6 F  Cvec=[0.3125, 6.2500e-02] uF  Vvec=[0, 600] V  CV_table_symmetry=ee.enum.passive.capacitor.tableSymmetry.yes  f_vec=[1, 10] kHz  DFext_vec=[.8, 1.2]  enable_C_tol=ee.enum.toleranceApplication.none  averaging_period=0 s  C_tol=5  tol_distribution=ee.enum.toleranceDistribution.uniform  nSigma=4  r=1e-6 Ohm  g=0 1/Ohm  enable_operating_limits=ee.enum.enable.no  operating_limit_action=ee.enum.passive.reportOpLim.warn  max_working_voltage_range=[-25, 25] V  power_rating=1 W  enable_faults=ee.enum.enable.no  fault_action=simscape.enum.assert.action.none  Cscale_faulted=100  R_faulted=1e-3 Ohm  G_faulted=0 1/Ohm  tau_fault=1e-3 s  fault_trigger=ee.enum.faults.faultTrigger.temporal  t_fault=1 s  max_permissible_voltage_range=[-100, 100] V  t_fail_on_voltage=1 s  i_specify=off  i_priority=None  i=0 A  i_nominal_specify=off  i_nominal_unit=A  i_nominal_value=1  v_specify=off  v_priority=None  v=0 V  v_nominal_specify=off  v_nominal_unit=V  v_nominal_value=1  vc_specify=off  vc_priority=High  vc=0 V  vc_nominal_specify=off  vc_nominal_unit=V  vc_nominal_value=1
  DC Voltage Source1 : ee_lib/Additional Components/SPICE Sources/DC Voltage Source  DC=570 V
  Demux : Demux  Outputs=6
  Diode{1..6} (6 alike) : ee_lib/Semiconductors & Converters/Diode  ModelType=ee.enum.diode.modelType.pwl  TableType=ee.enum.diode.tableType.IfMat  IfMat=[.07, .12, .19, 1.75, 4.24, 7.32, 11.2; .16, .3, .72, 2.14, 5.02, 8.35, 13.12] A  VfMat=[.9, 1.15, 1.25, 1.5, 1.75, 2.17, 2.6, 2.85; .58, .68, .75, 1.1, 1.38, 1.77, 2.27, 2.7] V  TjVec=[25, 125] degC  VfVec=[.5, .7, .9, 1.3, 1.7, 2.1, 2.5] V  IfVec=[.1, .2, .5, 1, 2, 4, 7, 10] A  Vf=0.6 V  Ron=0.3 Ohm  Goff=1e-8 S  prmExp=ee.enum.diode.expParam.useTwo  I12=[.0137, .545] A  V12=[.6, .7] V  RS=0 Ohm  Tmeas=25 degC  IS=1e-12 A  ec=1  I1=0.0137 A  V1=0.6 V  N_series=1  N_parallel=1  ZenerEnable=false  Rz=0.3 Ohm  BV=inf V  C_param=ee.enum.diode.capParam.fixed  CJ=0 pF  CJ0=5 pF  Vvec=[.1, 10, 100] V  Cvec=[3.5, 1, .4] pF  VJ=1 V  Mgrad=0.5  FC=0.5  Q_param=ee.enum.diode.recoveryParam.off  iRM=-7.15 A  iF=4 A  didt=-750 A/us  trr_factor=3  trr=115 ns  Qrr=150 nA*s  Vr=-600 V  Ls=150 nH  Erec=0.03 J  TT=50 ns  tau=100 ns  T_param=ee.enum.diode.temperatureParam.off  Tdevice=25 degC  I1_T2=0.245 A  V1_T2=0.5 V  IS_T2=1.25e-7 A  Tmeas2=125 degC  XTI_param=ee.enum.diode.xtiParam.pn  XTI=3  EG_param=ee.enum.diode.egapParam.material_si  EG=1.11 eV  dBVdT=0 V/K  enable_faults=simscape.enum.onoff.off  fault_action=simscape.enum.assert.action.none  fault_types=ee.enum.diode.faults.open  tau_fault=1e-3 s  IfMat_faulted=[.07, .12, .19, 1.75, 4.24, 7.32, 11.2; .16, .3, .72, 2.14, 4.02, 6.35, 9.12] A  VfMat_faulted=[.9, 1.15, 1.25, 1.5, 1.75, 2.17, 2.6, 2.85; .58, .68, .75, 1.1, 1.38, 1.77, 2.27, 2.7] V  VfVec_faulted=[.5, .7, .9, 1.3, 1.7, 2.1, 2.5] V  IfVec_faulted=[.1, .2, .5, 1, 2, 4, 7, 10] A  Ropen_faulted=1000 Ohm  Gshort_faulted=1000 1/Ohm  Vf_faulted=0.6 V  Ron_faulted=0.3 Ohm  Goff_faulted=1e-8 S  I12_faulted=[.0137, .545] A  V12_faulted=[.6, .7] V  IS_faulted=1e-12 A  ec_faulted=1  I1_faulted=0.0137 A  V1_faulted=0.6 V  RS_faulted=0 Ohm  Rz_faulted=0.3 Ohm  BV_faulted=inf V  Cscale_faulted=100  fault_trigger=ee.enum.faults.faultTrigger.temporal  t_fault=inf s  max_permissible_voltage=inf V  n_fail_on_voltage=1  max_permissible_current=inf A  t_fail_on_current=1 s  max_permissible_dVdt=inf V/s  enable_fault_input=simscape.enum.onoff.off  i_specify=off  i_priority=None  i=0 A  i_nominal_specify=off  i_nominal_unit=A  i_nominal_value=1  v_specify=off  v_priority=None  v=0 V  v_nominal_specify=off  v_nominal_unit=V  v_nominal_value=1  v_capacitor_specify=off  v_capacitor_priority=None  v_capacitor=0 V  v_capacitor_nominal_specify=off  v_capacitor_nominal_unit=V  v_capacitor_nominal_value=1  faulted_specify=off  faulted_priority=None  faulted=0  faulted_nominal_specify=off  faulted_nominal_unit=1  faulted_nominal_value=1  i_diode_specify=off  i_diode_priority=None  i_diode=0 A  i_diode_nominal_specify=off  i_diode_nominal_unit=A  i_diode_nominal_value=1  v_diode_specify=off  v_diode_priority=None  v_diode=0 V  v_diode_nominal_specify=off  v_diode_nominal_unit=V  v_diode_nominal_value=1  i_capacitor_specify=off  i_capacitor_priority=None  i_capacitor=0 A  i_capacitor_nominal_specify=off  i_capacitor_nominal_unit=A  i_capacitor_nominal_value=1  power_dissipated_specify=off  power_dissipated_priority=None  power_dissipated=0 W  power_dissipated_nominal_specify=off  power_dissipated_nominal_unit=W  power_dissipated_nominal_value=1  fidelity_level=ee.enum.diode.fidelity.includeChargeDyn  rec_loss_model=ee.enum.diode.reverseRecoveryModel.fixed  ErecVal=0 J  scaleWithIandV=true  ErecMat=zeros(2, 3) J  TjrecVec=[298.15, 398.15] K  IfrecVec=[.1, 1, 10] A  IrecVal=10 A  VrecVal=10 V  tFilter=1 / 1000 / 100 s  max_permissible_temperature=inf K  t_fail_on_temperature=1 s  thermal_network_parameterization=ee.enum.thermalNetworkTopology.junctionCase  Rth=[0, 10] K/W  Rth_Cauer=[1, 3, 10] K/W  Rth_Foster=[4, 6] K/W  thermal_mass_parameterization=ee.enum.thermalNetwork.timeconstant  thermal_mass=[0, 1] J/K  thermal_mass_Cauer=[.1, .3, 1] J/K  thermal_mass_Foster=[1.5, 3] J/K  thermal_time_constant=[0, 10] s  thermal_time_constant_Cauer=[1, 3, 10] s  thermal_time_constant_Foster=[6, 18] s  thermal_mass_initial_temperatures=[25, 25] degC  thermal_mass_initial_temperatures_Cauer=[25, 25, 25] degC  junction_thermal_mass=0.01 J/K  Tvec_initial_Foster=[25, 25, 25, 25] degC  no_thermal_network=0  junction_temperature_specify=off  junction_temperature_priority=None  junction_temperature=25 degC  junction_temperature_nominal_specify=off  junction_temperature_nominal_unit=degC  junction_temperature_nominal_value=1
  Electrical Reference : fl_lib/Electrical/Electrical Elements/Electrical Reference
  IGBT (Ideal, Switching){,1..5} (6 alike) : ee_lib/Semiconductors & Converters/IGBT (Ideal, Switching)  port_option=ee.enum.controlport.ps  Vf=0.8 V  Ron=0.0001 Ohm  Goff=1e-5 1/Ohm  Vth=6 V  diode_param=ee.enum.converters.protectiondiode.none  diode_Vf=0.8 V  diode_Ron=0.001 Ohm  diode_Goff=1e-5 1/Ohm  diode_C=50e-9 F  diode_iRM=-235 A  diode_iF=300 A  diode_idot=-50 A/us  diode_trr_param=ee.enum.converters.diodeReverseParam.trr_factor  diode_trr_factor=3  diode_trr=15 us  diode_Qrr=1500 s*uA  ice_specify=off  ice_priority=None  ice=0 A  ice_nominal_specify=off  ice_nominal_unit=A  ice_nominal_value=1  vce_specify=off  vce_priority=None  vce=0 V  vce_nominal_specify=off  vce_nominal_unit=V  vce_nominal_value=1  vge_specify=off  vge_priority=None  vge=0 V  vge_nominal_specify=off  vge_nominal_unit=V  vge_nominal_value=1  thermal_loss_option=ee.enum.converters.thermalLossOption.constantvalues  Von_data=[0, .1, .6, .8, 1, 1.3, 1.6, 2, 2.4; 0, .1, .7, 1, 1.2, 1.5, 1.9, 2.4, 2.8] V  Tj=[298.15, 398.15] K  Iout_data=[0, .1, 1, 5, 10, 20, 40, 70, 100] A  Eon_data=[0, .0024, .024, .12, .2, .48, 1.04, 2.16, 3.24; 0, .003, .03, .15, .25, .6, 1.3, 2.7, 4.05] * 1e-3 J  Eoff_data=[0, .0007, .0066, .033, .066, .17, .33, .83, 1.5; 0, .001, .01, .05, .1, .25, .5, 1.2, 2.2] * 1e-3 J  Eon_data_3D=[zeros(2, 9, 3)] J  Eoff_data_3D=[zeros(2, 9, 3)] J  Tj_loss=[298.15, 398.15] K  Iout_data_loss=[0, .1, 1, 5, 10, 20, 40, 70, 100] A  tabulateWithVce=false  Vce_loss=[0, 150, 300] V  Eon_scalar=22.86e-3 J  Eoff_scalar=17.14e-3 J  Voff=300 V  Iout_scalar=600 A  useCurrentFromPreviousCycle=false  useVoltageFromPreviousCycle=false  diodeModelType=ee.enum.converters.diodeModelType.pwl  diodeTableType=ee.enum.diode.tableType.IfMat  diode_IfMat=[.07, .12, .19, 1.75, 4.24, 7.32, 11.2; .16, .3, .72, 2.14, 4.02, 6.35, 9.12] A  diode_VfMat=[.9, 1.15, 1.25, 1.5, 1.75, 2.17, 2.6, 2.85; .58, .68, .75, 1.1, 1.38, 1.77, 2.27, 2.7] V  diode_TjVec=[25, 125] degC  diode_VfVec=[.5, .7, .9, 1.3, 1.7, 2.1, 2.5] V  diode_IfVec=[.1, .2, .5, 1, 2, 4, 7, 10] A  diode_Vr=-600 V  diode_Ls=150 nH  diode_Erec=0.03 J  diode_rec_loss_model=ee.enum.diode.reverseRecoveryModel.fixed  diode_ErecVal=0 J  diode_scaleWithIandV=true  diode_ErecMat=zeros(2, 3) J  diode_TjrecVec=[298.15, 398.15] K  diode_IfrecVec=[.1, 1, 10] A  diode_IrecVal=10 A  diode_VrecVal=10 V  diode_tFilter=1 / 1000 / 100 s  thermal_network_parameterization=ee.enum.thermalNetworkTopology.external  Rth=[.08, .5] K/W  Rth_Cauer=[.08, .1, .5] K/W  Rth_Foster=[.08, .14, .22, .16] K/W  thermal_mass_parameterization=ee.enum.thermalNetwork.timeconstant  thermal_mass=[.01, .5] J/K  thermal_mass_Cauer=[.01, .1, .5] J/K  thermal_mass_Foster=[.001, .005, .05, .5] J/K  thermal_time_constant=[.001, .2] s  thermal_time_constant_Cauer=[.001, .1, .2] s  thermal_time_constant_Foster=[7e-05, .0007, .01, .08] s  thermal_mass_initial_temperatures=[25, 25] degC  thermal_mass_initial_temperatures_Cauer=[25, 25, 25] degC  junction_thermal_mass=0.01 J/K  Tvec_initial_Foster=[25, 25, 25, 25] degC  no_thermal_network=0  junction_temperature_specify=off  junction_temperature_priority=None  junction_temperature=25 degC  junction_temperature_nominal_specify=off  junction_temperature_nominal_unit=degC  junction_temperature_nominal_value=1  Qj_specify=off  Qj_priority=None  Qj=0 W  Qj_nominal_specify=off  Qj_nominal_unit=W  Qj_nominal_value=1  accumulatedSwitchingLosses_specify=off  accumulatedSwitchingLosses_priority=None  accumulatedSwitchingLosses=0 J
  Simulink-PS Converter{,1..5} (6 alike) : nesl_utility/Simulink-PS Converter  PhysicalDomain=network_engine_domain  SubClassName=ps_input  LeftPortType=input  RightPortType=output  PseudoPeriodic=off  Frequencies=[]  NoiseDistribution=none  NoiseParameters=[]  Unit=1  AffineConversion=off  FilteringAndDerivatives=provide  SimscapeFilterOrder=1  InputFilterTimeConstant=0.001  UdotUserProvided=0
  Conn4 : PMIOPort  Side=Right
  Conn5 : PMIOPort  Port=2  Side=Right
  Conn6 : PMIOPort  Port=3  Side=Right
  wires:
  [PWM_UL] -> Simulink-PS Converter1/1
  [PWM_UH] -> Simulink-PS Converter/1
  Demux/5 -> [PWM_WH]
  PWM/1 -> Demux/1
  Demux/4 -> [PWM_VL]
  Demux/1 -> [PWM_UH]
  Demux/2 -> [PWM_UL]
  Demux/6 -> [PWM_WL]
  Demux/3 -> [PWM_VH]
  [PWM_VH] -> Simulink-PS Converter3/1
  [PWM_VL] -> Simulink-PS Converter2/1
  [PWM_WH] -> Simulink-PS Converter4/1
  [PWM_WL] -> Simulink-PS Converter5/1
  connections:
  Diode4/RConn1 -- "IGBT (Ideal, Switching)5"/RConn1 -- Diode3/LConn1 -- "IGBT (Ideal, Switching)4"/RConn2 -- Conn6/RConn1
  Electrical Reference/LConn1 -- Capacitor/RConn1 -- Capacitor1/LConn1
  Simulink-PS Converter4/RConn1 -- "IGBT (Ideal, Switching)4"/LConn1
  Simulink-PS Converter/RConn1 -- "IGBT (Ideal, Switching)"/LConn1
  Diode6/RConn1 -- "IGBT (Ideal, Switching)1"/RConn1 -- Diode1/LConn1 -- "IGBT (Ideal, Switching)"/RConn2 -- Conn4/RConn1
  Diode3/RConn1 -- "IGBT (Ideal, Switching)4"/RConn1 -- Diode2/RConn1 -- "IGBT (Ideal, Switching)2"/RConn1 -- Diode1/RConn1 -- "IGBT (Ideal, Switching)"/RConn1 -- Capacitor/LConn1 -- DC Voltage Source1/LConn1
  Diode5/RConn1 -- "IGBT (Ideal, Switching)3"/RConn1 -- Diode2/LConn1 -- "IGBT (Ideal, Switching)2"/RConn2 -- Conn5/RConn1
  DC Voltage Source1/RConn1 -- Diode6/LConn1 -- Diode5/LConn1 -- Diode4/LConn1 -- "IGBT (Ideal, Switching)5"/RConn2 -- "IGBT (Ideal, Switching)3"/RConn2 -- "IGBT (Ideal, Switching)1"/RConn2 -- Capacitor1/RConn1
  Simulink-PS Converter3/RConn1 -- "IGBT (Ideal, Switching)2"/LConn1
  "IGBT (Ideal, Switching)5"/LConn1 -- Simulink-PS Converter5/RConn1
  Simulink-PS Converter2/RConn1 -- "IGBT (Ideal, Switching)3"/LConn1
  Simulink-PS Converter1/RConn1 -- "IGBT (Ideal, Switching)1"/LConn1

== system PhyMtrCtrl/Subsystem2 ==
  Bus Creator : BusCreator  Inputs=6
  Bus Creator1 : BusCreator  Inputs=3
  Current Measurement : spsCurrentMeasurementLib/Current Measurement  PhasorSimulation=off  OutputType=Complex  PSBequivalent=0
  Current Measurement1 : spsCurrentMeasurementLib/Current Measurement  PhasorSimulation=off  OutputType=Complex  PSBequivalent=0
  Current Measurement2 : spsCurrentMeasurementLib/Current Measurement  PhasorSimulation=off  OutputType=Complex  PSBequivalent=0
  U : spsSeriesRLCBranchLib/Series RLC Branch  LConnTagsString=__new0  RConnTagsString=__new0  BranchType=RL  Resistance=4.5e-2  Inductance=1.35e-4  SetiL0=off  InitialCurrent=0  Capacitance=1e-6  Setx0=off  InitialVoltage=0  Measurements=None
  V : spsSeriesRLCBranchLib/Series RLC Branch  LConnTagsString=__new0  RConnTagsString=__new0  BranchType=RL  Resistance=4.5e-2  Inductance=1.35e-4  SetiL0=off  InitialCurrent=0  Capacitance=1e-6  Setx0=off  InitialVoltage=0  Measurements=None
  Voltage Measurement{1..6} (6 alike) : spsVoltageMeasurementLib/Voltage Measurement  PhasorSimulation=off  OutputType=Complex  PSBequivalent=0
  W : spsSeriesRLCBranchLib/Series RLC Branch  LConnTagsString=__new0  RConnTagsString=__new0  BranchType=RL  Resistance=4.5e-2  Inductance=1.35e-4  SetiL0=off  InitialCurrent=0  Capacitance=1e-6  Setx0=off  InitialVoltage=0  Measurements=None
  A : PMIOPort  Side=Left
  B : PMIOPort  Port=2  Side=Left
  C : PMIOPort  Port=3  Side=Left
  Voltage M : Outport
  Current M : Outport  Port=2
  wires:
  Bus Creator1/1 -> Current M/1
  Current Measurement2/1 -> Bus Creator1/3  "Ic"
  Current Measurement1/1 -> Bus Creator1/2  "Ib"
  Current Measurement/1 -> Bus Creator1/1  "Ia"
  Bus Creator/1 -> Voltage M/1
  Voltage Measurement2/1 -> Bus Creator/4  "Vb"
  Voltage Measurement6/1 -> Bus Creator/6  "Vc"
  Voltage Measurement1/1 -> Bus Creator/5  "Vac"
  Voltage Measurement3/1 -> Bus Creator/1  "Va"
  Voltage Measurement4/1 -> Bus Creator/2  "Vab"
  Voltage Measurement5/1 -> Bus Creator/3  "Vbc"
  connections:
  Current Measurement2/LConn1 -- C/RConn1
  B/RConn1 -- Current Measurement1/LConn1
  Current Measurement/LConn1 -- A/RConn1
  Voltage Measurement4/LConn1 -- Voltage Measurement3/LConn1 -- U/LConn1 -- Current Measurement/RConn1 -- Voltage Measurement1/LConn1
  V/RConn1 -- Voltage Measurement2/LConn2 -- W/RConn1 -- Voltage Measurement6/LConn2 -- Voltage Measurement3/LConn2 -- U/RConn1
  V/LConn1 -- Current Measurement1/RConn1 -- Voltage Measurement2/LConn1 -- Voltage Measurement4/LConn2 -- Voltage Measurement5/LConn1
  W/LConn1 -- Current Measurement2/RConn1 -- Voltage Measurement6/LConn1 -- Voltage Measurement5/LConn2 -- Voltage Measurement1/LConn2

== system PhyMtrCtrl/TqCtrl ==
  TqRef : Inport
  TqFb : Inport  Port=2
  Sat : Inport  Port=3
  Scope5 : Scope  NumInputPorts=2
  Subsystem1 : Subsystem
  CurSet : Outport
  wires:
  Sat/1 -> Subsystem1/3(Sat)
  TqRef/1 -> Subsystem1/1(Ref), Scope5/1
  TqFb/1 -> Subsystem1/2(Fbk), Scope5/2
  Subsystem1/1(PIOut) -> CurSet/1  "TqPIOut"

== system PhyMtrCtrl/CurLpCtrl/ClarkeTF ==
  CurA : Inport  OutDataTypeStr=fixdt(1,32,31)
  CurB : Inport  Port=2  OutDataTypeStr=fixdt(1,32,31)
  Add : Sum  Inputs=+++  OutDataTypeStr=fixdt(1,32,31)
  Constant : Constant  Value=C_MATH_OneOverSqrtThree_s32n31_Null  OutDataTypeStr=fixdt(1,32,31)
  Data Type Conversion : DataTypeConversion  OutDataTypeStr=fixdt(1,16,15)  SaturateOnIntegerOverflow=off  RndMeth=Floor
  Data Type Conversion1 : DataTypeConversion  OutDataTypeStr=fixdt(1,16,15)  SaturateOnIntegerOverflow=off  RndMeth=Floor
  Data Type Conversion2 : DataTypeConversion  SaturateOnIntegerOverflow=off  RndMeth=Floor
  Product : Product
  I_alpha : Outport
  I_beta : Outport  Port=2
  wires:
  Add/1 -> Data Type Conversion/1
  CurB/1 -> Add/3, Add/2
  CurA/1 -> I_alpha/1, Add/1
  Product/1 -> Data Type Conversion2/1
  Constant/1 -> Data Type Conversion1/1
  Data Type Conversion/1 -> Product/1
  Data Type Conversion1/1 -> Product/2
  Data Type Conversion2/1 -> I_beta/1

== system PhyMtrCtrl/CurLpCtrl/CurCal ==
  CurU : Inport  OutDataTypeStr=fixdt(1,32,31)
  CurW : Inport  Port=2  OutDataTypeStr=fixdt(1,32,31)
  Scope : Scope  NumInputPorts=3
  Subtract : Sum  Inputs=--  OutDataTypeStr=fixdt(1,32,31)
  CurA : Outport
  CurB : Outport  Port=2
  CurC : Outport  Port=3
  wires:
  CurU/1 -> Subtract/1, Scope/1, CurA/1  "Ia"
  CurW/1 -> Subtract/2, Scope/3, CurC/1
  Subtract/1 -> Scope/2, CurB/1  "Ib"

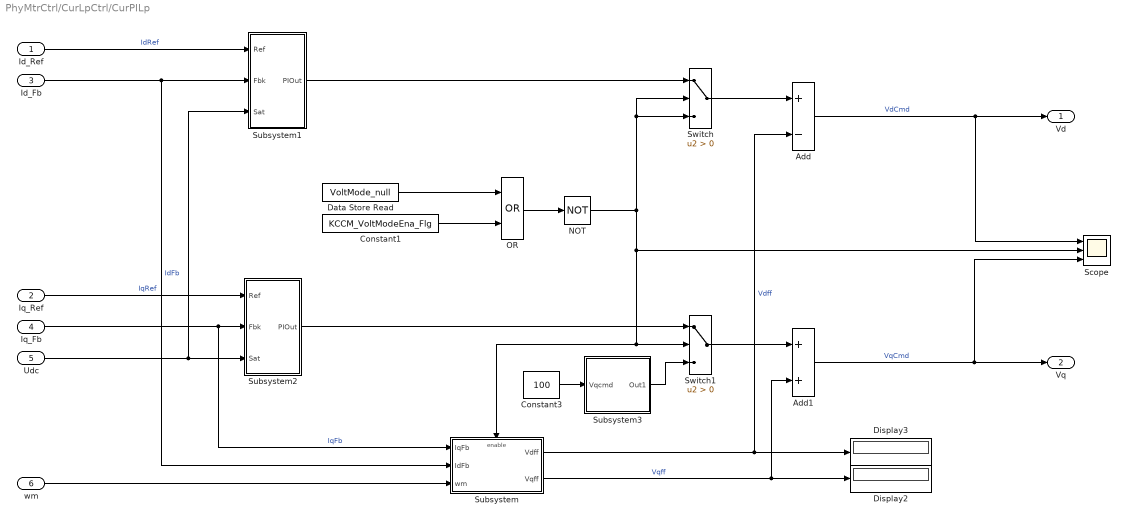
== system PhyMtrCtrl/CurLpCtrl/CurPILp ==
  Id_Ref : Inport  OutDataTypeStr=fixdt(1,32,31)
  Iq_Ref : Inport  Port=2  OutDataTypeStr=fixdt(1,32,31)
  Id_Fb : Inport  Port=3  OutDataTypeStr=fixdt(1,32,31)
  Iq_Fb : Inport  Port=4  OutDataTypeStr=fixdt(1,32,31)
  Udc : Inport  Port=5  OutDataTypeStr=fixdt(0,32,32)
  wm : Inport  Port=6  OutDataTypeStr=fixdt(1,32,31)
  Add : Sum  Inputs=+-  OutDataTypeStr=fixdt(1,32,31)
  Add1 : Sum  OutDataTypeStr=fixdt(1,32,31)
  Constant1 : Constant  Value=KCCM_VoltModeEna_Flg  OutDataTypeStr=boolean
  Constant3 : Constant  Value=100  OutDataTypeStr=fixdt(0,32,25)
  Data Store Read : DataStoreRead  DataStoreName=VoltMode_null  IndexOptions=Index vector (dialog)  Indices=1  OutputSizes=1
  Display2 : Display
  Display3 : Display
  NOT : Logic  Operator=NOT  AllPortsSameDT=off  OutDataTypeStr=boolean
  OR : Logic  Operator=OR  AllPortsSameDT=off  OutDataTypeStr=boolean
  Scope : Scope  NumInputPorts=3
  Subsystem : Subsystem
  Subsystem1 : Subsystem
  Subsystem2 : Subsystem
  Subsystem3 : Subsystem
  Switch : Switch  Criteria=u2 > Threshold  OutDataTypeStr=fixdt(1,32,32)  SaturateOnIntegerOverflow=off  InputSameDT=off
  Switch1 : Switch  Criteria=u2 > Threshold  OutDataTypeStr=fixdt(1,32,31)  SaturateOnIntegerOverflow=off  InputSameDT=off
  Vd : Outport
  Vq : Outport  Port=2
  wires:
  Subsystem1/1(PIOut) -> Switch/1
  Iq_Ref/1 -> Subsystem2/1(Ref)  "IqRef"
  Id_Ref/1 -> Subsystem1/1(Ref)  "IdRef"
  Id_Fb/1 -> Subsystem/2(IdFb), Subsystem1/2(Fbk)  "IdFb"
  Iq_Fb/1 -> Subsystem2/2(Fbk), Subsystem/1(IqFb)  "IqFb"
  OR/1 -> NOT/1
  Switch/1 -> Add/1
  Switch1/1 -> Add1/1
  wm/1 -> Subsystem/3(wm)
  Subsystem/2(Vqff) -> Add1/2, Display2/1  "Vqff"
  Subsystem/1(Vdff) -> Add/2, Display3/1  "Vdff"
  Add1/1 -> Scope/3, Vq/1  "VqCmd"
  Add/1 -> Scope/1, Vd/1  "VdCmd"
  Udc/1 -> Subsystem2/3(Sat), Subsystem1/3(Sat)
  Subsystem2/1(PIOut) -> Switch1/1
  Subsystem3/1(Out1) -> Switch1/3
  Constant3/1 -> Subsystem3/1(Vqcmd)
  Data Store Read/1 -> OR/1
  Constant1/1 -> OR/2
  NOT/1 -> Scope/2, Subsystem/Enable, Switch1/2, Switch/3, Switch/2
